simulink model "ip_model"  (R2013a)
settings: Solver=ode45  StartTime=0.0  StopTime=10.0  RelTol=1e-3
values from neighbouring files (symbols this model uses):
  a1 = 6.20e+000    (= 6.2)    [adip_para.m]
  ac = 6.25e+000    (= 6.25)    [cdip_para.m]
  alpha2 = J2 + m2*l2^2    (= 0.0045564)    [adip_para.m]
  alpha3 = m2*L1*l2    (= 0.00424944)    [adip_para.m]
  alpha5 = m2*l2*g    (= 0.1836432)    [adip_para.m]
  b1 = 1.58e+001    (= 15.8)    [adip_para.m]
  bc = 4.36e+000    (= 4.36)    [cdip_para.m]
  g = 9.81e+000    (= 9.81)    [adip_para.m]    (also in cdip_para.m)
  Jp = 1.59e-003    (= 0.00159)    [cdip_para.m]
  lp = 2.30e-001    (= 0.23)    [cdip_para.m]
  mp = 1.07e-001    (= 0.107)    [cdip_para.m]
  mu2 = 1.01e-004    (= 0.000101)    [adip_para.m]
  mup = 2.35e-004    (= 0.000235)    [cdip_para.m]
undefined symbols (not defined in the file or in its folder): dtheta1_0, dtheta2_0, dtheta_0, dz_0, theta1_0, theta2_0, theta_0, z_0
settings Model: Creator=kawata  LastModifiedBy=kawata
settings DataIOCC: SignalLoggingSaveFormat=ModelDataLogs
settings OptimizationCC: ExpressionDepthLimit=2147483647
settings DebuggingCC: FcnCallInpInsideContextMsg=UseLocalSettings
settings GRTTargetCC: CombineOutputUpdateFcns=off  GRTInterface=on

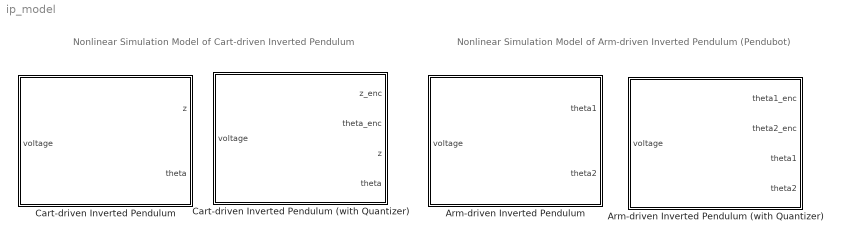
== system ip_model ==
  note: Nonlinear Simulation Model
      | of Cart-driven Inverted Pendulum
  note: Nonlinear Simulation Model
      | of Arm-driven Inverted Pendulum (Pendubot)
  Arm-driven Inverted Pendulum : Subsystem
      mask Display: image(imread('adip.jpg'),'center')
  Arm-driven Inverted Pendulum (with Quantizer) : Subsystem
      mask Display: image(imread('adip_photo.jpg'),'center')
  Cart-driven Inverted Pendulum : Subsystem
      mask Display: image(imread('cdip.jpg'),'center')
  Cart-driven Inverted Pendulum (with Quantizer) : Subsystem
      mask Display: image(imread('cdip_photo.jpg'),'center')

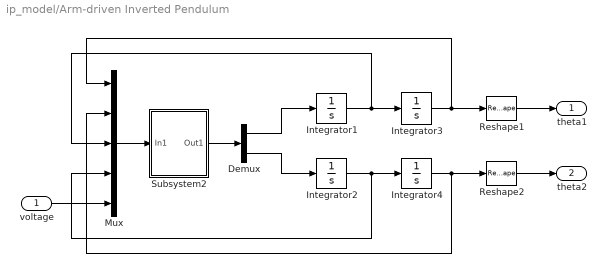
== system ip_model/Arm-driven Inverted Pendulum ==
  voltage : Inport
  Demux : Demux  Outputs=2
  Integrator1 : Integrator  InitialCondition=dtheta1_0
  Integrator2 : Integrator  InitialCondition=dtheta2_0
  Integrator3 : Integrator  InitialCondition=theta1_0
  Integrator4 : Integrator  InitialCondition=theta2_0
  Mux : Mux  Inputs=5
  Reshape1 : Reshape
  Reshape2 : Reshape
  Subsystem2 : Subsystem
  theta1 : Outport
  theta2 : Outport  Port=2
  wires:
  voltage/1 -> Mux/5
  Integrator4/1 -> Mux/2, Reshape2/1
  Integrator3/1 -> Mux/1, Reshape1/1
  Integrator2/1 -> Integrator4/1, Mux/4
  Integrator1/1 -> Integrator3/1, Mux/3
  Demux/2 -> Integrator2/1
  Demux/1 -> Integrator1/1
  Mux/1 -> Subsystem2/1(In1)
  Subsystem2/1(Out1) -> Demux/1
  Reshape2/1 -> theta2/1
  Reshape1/1 -> theta1/1

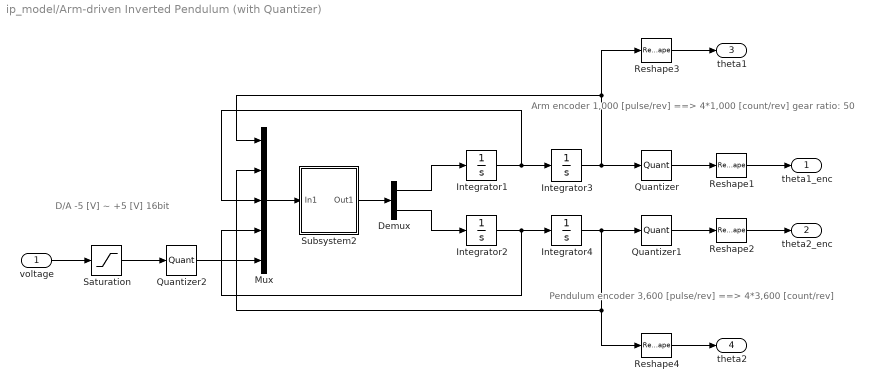
== system ip_model/Arm-driven Inverted Pendulum (with Quantizer) ==
  note: D/A
      |   -5 [V] ~ +5 [V]
      |  16bit
  note: Arm encoder
      |   1,000 [pulse/rev]  ==> 4*1,000 [count/rev]
      |   gear ratio: 50
  note: Pendulum encoder
      |   3,600 [pulse/rev]  ==> 4*3,600 [count/rev]
  voltage : Inport
  Demux : Demux  Outputs=2
  Integrator1 : Integrator  InitialCondition=dtheta1_0
  Integrator2 : Integrator  InitialCondition=dtheta2_0
  Integrator3 : Integrator  InitialCondition=theta1_0
  Integrator4 : Integrator  InitialCondition=theta2_0
  Mux : Mux  Inputs=5
  Quantizer : Quantizer  QuantizationInterval=2*pi/(4*1000*50)
  Quantizer1 : Quantizer  QuantizationInterval=2*pi/(4*3600)
  Quantizer2 : Quantizer  QuantizationInterval=10/2^(16)
  Reshape{1..4} (4 alike) : Reshape
  Saturation : Saturate  UpperLimit=5  LowerLimit=-5
  Subsystem2 : Subsystem
  theta1_enc : Outport
  theta2_enc : Outport  Port=2
  theta1 : Outport  Port=3
  theta2 : Outport  Port=4
  wires:
  Saturation/1 -> Quantizer2/1
  Quantizer1/1 -> Reshape2/1
  Quantizer/1 -> Reshape1/1
  voltage/1 -> Saturation/1
  Reshape1/1 -> theta1_enc/1
  Reshape2/1 -> theta2_enc/1
  Quantizer2/1 -> Mux/5
  Integrator4/1 -> Quantizer1/1, Mux/2, Reshape4/1
  Integrator3/1 -> Quantizer/1, Mux/1, Reshape3/1
  Integrator2/1 -> Mux/4, Integrator4/1
  Integrator1/1 -> Mux/3, Integrator3/1
  Demux/2 -> Integrator2/1
  Demux/1 -> Integrator1/1
  Mux/1 -> Subsystem2/1(In1)
  Subsystem2/1(Out1) -> Demux/1
  Reshape3/1 -> theta1/1
  Reshape4/1 -> theta2/1

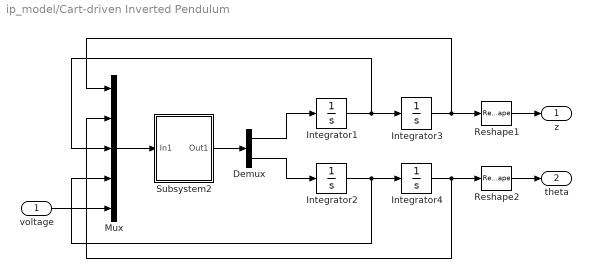
== system ip_model/Cart-driven Inverted Pendulum ==
  voltage : Inport
  Demux : Demux  Outputs=2
  Integrator1 : Integrator  InitialCondition=dz_0
  Integrator2 : Integrator  InitialCondition=dtheta_0
  Integrator3 : Integrator  InitialCondition=z_0
  Integrator4 : Integrator  InitialCondition=theta_0
  Mux : Mux  Inputs=5
  Reshape1 : Reshape
  Reshape2 : Reshape
  Subsystem2 : Subsystem
  z : Outport
  theta : Outport  Port=2
  wires:
  Subsystem2/1(Out1) -> Demux/1
  Mux/1 -> Subsystem2/1(In1)
  Demux/1 -> Integrator1/1
  Demux/2 -> Integrator2/1
  Integrator1/1 -> Mux/3, Integrator3/1
  Integrator2/1 -> Mux/4, Integrator4/1
  Integrator3/1 -> Reshape1/1, Mux/1
  Integrator4/1 -> Reshape2/1, Mux/2
  voltage/1 -> Mux/5
  Reshape1/1 -> z/1
  Reshape2/1 -> theta/1

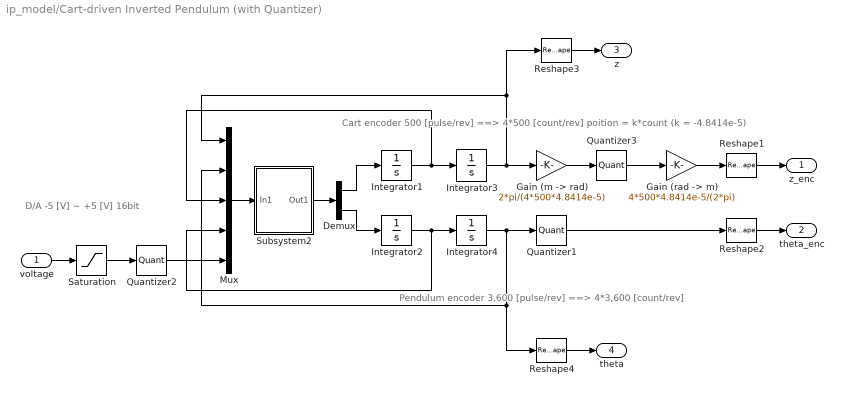
== system ip_model/Cart-driven Inverted Pendulum (with Quantizer) ==
  note: Pendulum encoder
      |   3,600 [pulse/rev]  ==> 4*3,600 [count/rev]
  note: D/A
      |   -5 [V] ~ +5 [V]
      |  16bit
  note: Cart encoder
      |   500 [pulse/rev]  ==> 4*500 [count/rev]
      |   poition = k*count  (k = -4.8414e-5)
  voltage : Inport
  Demux : Demux  Outputs=2
  "Gain (m -> rad)" : Gain  Gain=2*pi/(4*500*4.8414e-5)  SaturateOnIntegerOverflow=on  OutDataTypeStr=Inherit: Same as input  ParamDataTypeStr=Inherit: Same as input
  "Gain (rad -> m)" : Gain  Gain=4*500*4.8414e-5/(2*pi)  SaturateOnIntegerOverflow=on  OutDataTypeStr=Inherit: Same as input  ParamDataTypeStr=Inherit: Same as input
  Integrator1 : Integrator  InitialCondition=dz_0
  Integrator2 : Integrator  InitialCondition=dtheta_0
  Integrator3 : Integrator  InitialCondition=z_0
  Integrator4 : Integrator  InitialCondition=theta_0
  Mux : Mux  Inputs=5
  Quantizer1 : Quantizer  QuantizationInterval=2*pi/(4*3600)
  Quantizer2 : Quantizer  QuantizationInterval=10/2^(16)
  Quantizer3 : Quantizer  QuantizationInterval=2*pi/(4*500)
  Reshape{1..4} (4 alike) : Reshape
  Saturation : Saturate  UpperLimit=5  LowerLimit=-5
  Subsystem2 : Subsystem
  z_enc : Outport
  theta_enc : Outport  Port=2
  z : Outport  Port=3
  theta : Outport  Port=4
  wires:
  Reshape2/1 -> theta_enc/1
  Reshape1/1 -> z_enc/1
  "Gain (rad -> m)"/1 -> Reshape1/1
  Quantizer3/1 -> "Gain (rad -> m)"/1
  "Gain (m -> rad)"/1 -> Quantizer3/1
  voltage/1 -> Saturation/1
  Integrator4/1 -> Quantizer1/1, Mux/2, Reshape4/1
  Integrator3/1 -> "Gain (m -> rad)"/1, Mux/1, Reshape3/1
  Integrator2/1 -> Integrator4/1, Mux/4
  Integrator1/1 -> Integrator3/1, Mux/3
  Demux/2 -> Integrator2/1
  Demux/1 -> Integrator1/1
  Mux/1 -> Subsystem2/1(In1)
  Subsystem2/1(Out1) -> Demux/1
  Quantizer1/1 -> Reshape2/1
  Quantizer2/1 -> Mux/5
  Saturation/1 -> Quantizer2/1
  Reshape3/1 -> z/1
  Reshape4/1 -> theta/1

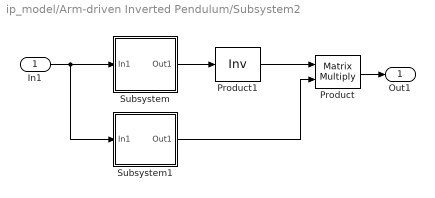
== system ip_model/Arm-driven Inverted Pendulum/Subsystem2 ==
  In1 : Inport
  Product : Product  Multiplication=Matrix(*)  SaturateOnIntegerOverflow=on  InputSameDT=on  OutDataTypeStr=Inherit: Same as first input
  Product1 : Product  Inputs=/  Multiplication=Matrix(*)  SaturateOnIntegerOverflow=on  InputSameDT=on  OutDataTypeStr=Inherit: Same as first input
  Subsystem : Subsystem
  Subsystem1 : Subsystem
  Out1 : Outport
  wires:
  Subsystem/1(Out1) -> Product1/1
  Product1/1 -> Product/1
  Subsystem1/1(Out1) -> Product/2
  In1/1 -> Subsystem/1(In1), Subsystem1/1(In1)
  Product/1 -> Out1/1

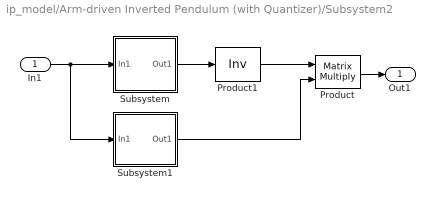
== system ip_model/Arm-driven Inverted Pendulum (with Quantizer)/Subsystem2 ==
  In1 : Inport
  Product : Product  Multiplication=Matrix(*)  SaturateOnIntegerOverflow=on  InputSameDT=on  OutDataTypeStr=Inherit: Same as first input
  Product1 : Product  Inputs=/  Multiplication=Matrix(*)  SaturateOnIntegerOverflow=on  InputSameDT=on  OutDataTypeStr=Inherit: Same as first input
  Subsystem : Subsystem
  Subsystem1 : Subsystem
  Out1 : Outport
  wires:
  Product/1 -> Out1/1
  In1/1 -> Subsystem1/1(In1), Subsystem/1(In1)
  Subsystem1/1(Out1) -> Product/2
  Product1/1 -> Product/1
  Subsystem/1(Out1) -> Product1/1

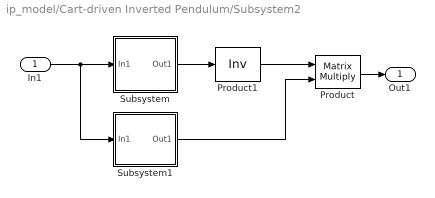
== system ip_model/Cart-driven Inverted Pendulum/Subsystem2 ==
  In1 : Inport
  Product : Product  Multiplication=Matrix(*)  SaturateOnIntegerOverflow=on  InputSameDT=on  OutDataTypeStr=Inherit: Same as first input
  Product1 : Product  Inputs=/  Multiplication=Matrix(*)  SaturateOnIntegerOverflow=on  InputSameDT=on  OutDataTypeStr=Inherit: Same as first input
  Subsystem : Subsystem
  Subsystem1 : Subsystem
  Out1 : Outport
  wires:
  Product/1 -> Out1/1
  In1/1 -> Subsystem1/1(In1), Subsystem/1(In1)
  Subsystem1/1(Out1) -> Product/2
  Product1/1 -> Product/1
  Subsystem/1(Out1) -> Product1/1

== system ip_model/Cart-driven Inverted Pendulum (with Quantizer)/Subsystem2 ==
  In1 : Inport
  Product : Product  Multiplication=Matrix(*)  SaturateOnIntegerOverflow=on  InputSameDT=on  OutDataTypeStr=Inherit: Same as first input
  Product1 : Product  Inputs=/  Multiplication=Matrix(*)  SaturateOnIntegerOverflow=on  InputSameDT=on  OutDataTypeStr=Inherit: Same as first input
  Subsystem : Subsystem
  Subsystem1 : Subsystem
  Out1 : Outport
  wires:
  Product/1 -> Out1/1
  In1/1 -> Subsystem1/1(In1), Subsystem/1(In1)
  Subsystem1/1(Out1) -> Product/2
  Product1/1 -> Product/1
  Subsystem/1(Out1) -> Product1/1

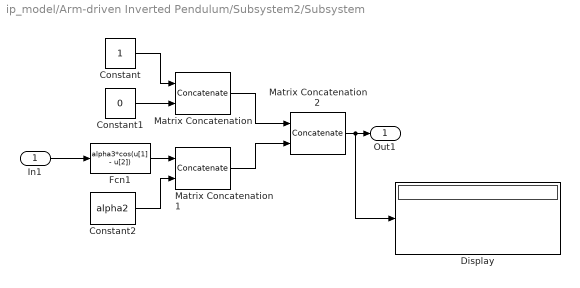
== system ip_model/Arm-driven Inverted Pendulum/Subsystem2/Subsystem ==
  In1 : Inport
  Constant : Constant
  Constant1 : Constant  Value=0
  Constant2 : Constant  Value=alpha2
  Display : Display
  Fcn1 : Fcn  Expr=alpha3*cos(u[1] - u[2])
  Matrix Concatenation : Concatenate  Mode=Multidimensional array  ConcatenateDimension=2
  Matrix Concatenation1 : Concatenate  Mode=Multidimensional array  ConcatenateDimension=2
  Matrix Concatenation2 : Concatenate  Mode=Multidimensional array
  Out1 : Outport
  wires:
  Constant2/1 -> Matrix Concatenation1/2
  Fcn1/1 -> Matrix Concatenation1/1
  In1/1 -> Fcn1/1
  Matrix Concatenation/1 -> Matrix Concatenation2/1
  Matrix Concatenation1/1 -> Matrix Concatenation2/2
  Matrix Concatenation2/1 -> Display/1, Out1/1
  Constant/1 -> Matrix Concatenation/1
  Constant1/1 -> Matrix Concatenation/2

== system ip_model/Arm-driven Inverted Pendulum/Subsystem2/Subsystem1 ==
  In1 : Inport
  Fcn1 : Fcn  Expr=- a1*u[3] + b1*u[5]
  Fcn2 : Fcn  Expr=alpha3*u[3]^2*sin(u[1] - u[2]) + alpha5*sin(u[2]) + mu2*u[3] - mu2*u[4]
  Matrix Concatenation1 : Concatenate  Mode=Multidimensional array
  Out1 : Outport
  wires:
  Fcn2/1 -> Matrix Concatenation1/2
  Fcn1/1 -> Matrix Concatenation1/1
  In1/1 -> Fcn2/1, Fcn1/1
  Matrix Concatenation1/1 -> Out1/1

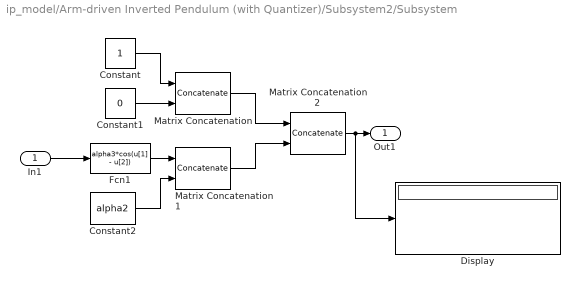
== system ip_model/Arm-driven Inverted Pendulum (with Quantizer)/Subsystem2/Subsystem ==
  In1 : Inport
  Constant : Constant
  Constant1 : Constant  Value=0
  Constant2 : Constant  Value=alpha2
  Display : Display
  Fcn1 : Fcn  Expr=alpha3*cos(u[1] - u[2])
  Matrix Concatenation : Concatenate  Mode=Multidimensional array  ConcatenateDimension=2
  Matrix Concatenation1 : Concatenate  Mode=Multidimensional array  ConcatenateDimension=2
  Matrix Concatenation2 : Concatenate  Mode=Multidimensional array
  Out1 : Outport
  wires:
  Constant1/1 -> Matrix Concatenation/2
  Constant/1 -> Matrix Concatenation/1
  Matrix Concatenation2/1 -> Out1/1, Display/1
  Matrix Concatenation1/1 -> Matrix Concatenation2/2
  Matrix Concatenation/1 -> Matrix Concatenation2/1
  In1/1 -> Fcn1/1
  Fcn1/1 -> Matrix Concatenation1/1
  Constant2/1 -> Matrix Concatenation1/2

== system ip_model/Arm-driven Inverted Pendulum (with Quantizer)/Subsystem2/Subsystem1 ==
  In1 : Inport
  Fcn1 : Fcn  Expr=- a1*u[3] + b1*u[5]
  Fcn2 : Fcn  Expr=alpha3*u[3]^2*sin(u[1] - u[2]) + alpha5*sin(u[2]) + mu2*u[3] - mu2*u[4]
  Matrix Concatenation1 : Concatenate  Mode=Multidimensional array
  Out1 : Outport
  wires:
  Matrix Concatenation1/1 -> Out1/1
  In1/1 -> Fcn1/1, Fcn2/1
  Fcn1/1 -> Matrix Concatenation1/1
  Fcn2/1 -> Matrix Concatenation1/2

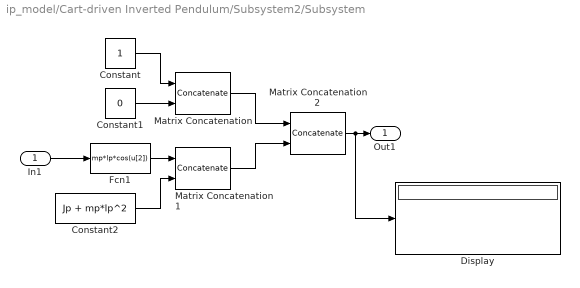
== system ip_model/Cart-driven Inverted Pendulum/Subsystem2/Subsystem ==
  In1 : Inport
  Constant : Constant
  Constant1 : Constant  Value=0
  Constant2 : Constant  Value=Jp + mp*lp^2
  Display : Display
  Fcn1 : Fcn  Expr=mp*lp*cos(u[2])
  Matrix Concatenation : Concatenate  Mode=Multidimensional array  ConcatenateDimension=2
  Matrix Concatenation1 : Concatenate  Mode=Multidimensional array  ConcatenateDimension=2
  Matrix Concatenation2 : Concatenate  Mode=Multidimensional array
  Out1 : Outport
  wires:
  Constant1/1 -> Matrix Concatenation/2
  Constant/1 -> Matrix Concatenation/1
  Matrix Concatenation2/1 -> Out1/1, Display/1
  Matrix Concatenation1/1 -> Matrix Concatenation2/2
  Matrix Concatenation/1 -> Matrix Concatenation2/1
  In1/1 -> Fcn1/1
  Fcn1/1 -> Matrix Concatenation1/1
  Constant2/1 -> Matrix Concatenation1/2

== system ip_model/Cart-driven Inverted Pendulum/Subsystem2/Subsystem1 ==
  In1 : Inport
  Fcn1 : Fcn  Expr=- ac*u[3] + bc*u[5]
  Fcn2 : Fcn  Expr=mp*lp*g*sin(u[2]) - mup*u[4]
  Matrix Concatenation1 : Concatenate  Mode=Multidimensional array
  Out1 : Outport
  wires:
  Matrix Concatenation1/1 -> Out1/1
  In1/1 -> Fcn1/1, Fcn2/1
  Fcn1/1 -> Matrix Concatenation1/1
  Fcn2/1 -> Matrix Concatenation1/2

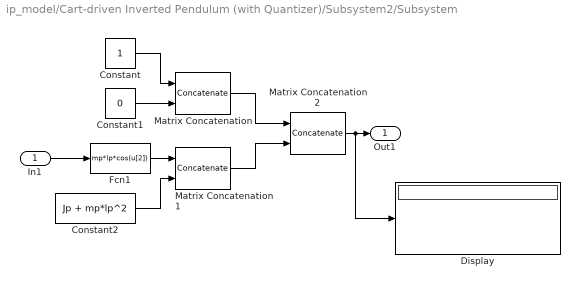
== system ip_model/Cart-driven Inverted Pendulum (with Quantizer)/Subsystem2/Subsystem ==
  In1 : Inport
  Constant : Constant
  Constant1 : Constant  Value=0
  Constant2 : Constant  Value=Jp + mp*lp^2
  Display : Display
  Fcn1 : Fcn  Expr=mp*lp*cos(u[2])
  Matrix Concatenation : Concatenate  Mode=Multidimensional array  ConcatenateDimension=2
  Matrix Concatenation1 : Concatenate  Mode=Multidimensional array  ConcatenateDimension=2
  Matrix Concatenation2 : Concatenate  Mode=Multidimensional array
  Out1 : Outport
  wires:
  Constant1/1 -> Matrix Concatenation/2
  Constant/1 -> Matrix Concatenation/1
  Matrix Concatenation2/1 -> Out1/1, Display/1
  Matrix Concatenation1/1 -> Matrix Concatenation2/2
  Matrix Concatenation/1 -> Matrix Concatenation2/1
  In1/1 -> Fcn1/1
  Fcn1/1 -> Matrix Concatenation1/1
  Constant2/1 -> Matrix Concatenation1/2

== system ip_model/Cart-driven Inverted Pendulum (with Quantizer)/Subsystem2/Subsystem1 ==
  In1 : Inport
  Fcn1 : Fcn  Expr=- ac*u[3] + bc*u[5]
  Fcn2 : Fcn  Expr=mp*lp*g*sin(u[2]) - mup*u[4]
  Matrix Concatenation1 : Concatenate  Mode=Multidimensional array
  Out1 : Outport
  wires:
  Matrix Concatenation1/1 -> Out1/1
  In1/1 -> Fcn1/1, Fcn2/1
  Fcn1/1 -> Matrix Concatenation1/1
  Fcn2/1 -> Matrix Concatenation1/2
